simulink model "sdl_testbed"  (R2022b)
settings: Solver=VariableStepAuto  StartTime=0.0  StopTime=5  RelTol=1e-3  AbsTol=1e-3  EnableMultiTasking=on
PreLoadFcn:
  | MFormulaCoeff.DryTarmac = [10 1.9 1 0.97];
  | MFormulaCoeff.WetTarmac = [12 2.3 0.82 1];
  | MFormulaCoeff.Snow         = [5 2 0.3 1];
  | MFormulaCoeff.Ice            = [4 2 0.1 1];
libraries: sdl_lib x22, nesl_utility x9, fl_ps_legacy_lib x5, fl_lib x4, simulink x1
(part 1 of 3)
CloseFcn:
  | try,close(h1_sdl_vehicle_4wd_testbed),end
  | clear h1_sdl_vehicle_4wd_testbed
  | try,close(h2_sdl_vehicle_4wd_testbed),end
  | clear h2_sdl_vehicle_4wd_testbed
  | try,close(h3_sdl_vehicle_4wd_testbed),end
  | clear h3_sdl_vehicle_4wd_testbed
  | 
  | clear simlog_sdl_vehicle_4wd_testbed
  | clear logsout_sdl_vehicle_4wd_testbed
Description:
  | Four-Wheel Drive Testbed
settings Model: PacingRate=0.110000  Creator=The MathWorks, Inc.  LastModifiedBy=jc790999
settings SolverCC: AutoScaleAbsTol=off  MaxConsecutiveMinStep=2  AlgebraicLoopSolver=TrustRegion
settings DataIOCC: LimitDataPoints=on  MaxDataPoints=10000  SaveTime=off  ReturnWorkspaceOutputs=off  SignalLoggingName=logsout_sdl_vehicle_4wd_testbed
settings OptimizationCC: LifeSpan=inf
settings DebuggingCC: UnconnectedInputMsg=warning  UnconnectedOutputMsg=warning  UnconnectedLineMsg=warning  SFUnexpectedBacktrackingDiag=warning  SFNoUnconditionalDefaultTransitionDiag=warning  SFExecutionAtInitializationDiag=none  SFMachineParentedDataDiag=warning  ArithmeticOperatorsInVariantConditions=warning
settings HardwareCC: ProdBitPerPointer=32  ProdBitPerSizeT=32  ProdBitPerPtrDiffT=32  ProdLargestAtomicFloat=None  ProdIntDivRoundTo=Undefined  ProdEndianess=Unspecified  ProdWordSize=32  ProdHWDeviceType=32-bit Generic
settings ModelReferenceCC: EnableRefExpFcnMdlSchedulingChecks=on  PropagateSignalLabelsOutOfModel=off
settings SFSimCC: SimUseLocalCustomCode=off  CustomCodeUndefinedFunction=UseInterfaceOnly
settings RTWCC: RTWUseLocalCustomCode=off  DLArmComputeVersion=19.05
settings CodeAppCC: StateflowObjectComments=on
settings GRTTargetCC: TargetLangStandard=C89/C90 (ANSI)
settings ConfigComp: CovMetricSettings=dw  CovSaveCumulativeToWorkspaceVar=on  CovSaveSingleToWorkspaceVar=on  CovExternalEMLEnable=off  CovSFcnEnable=off
settings SimscapeCC: SimscapeLogType=all  SimscapeLogSimulationStatistics=on  SimscapeLogName=simlog_sdl_vehicle_4wd_testbed  SimscapeLogDataHistory=10000

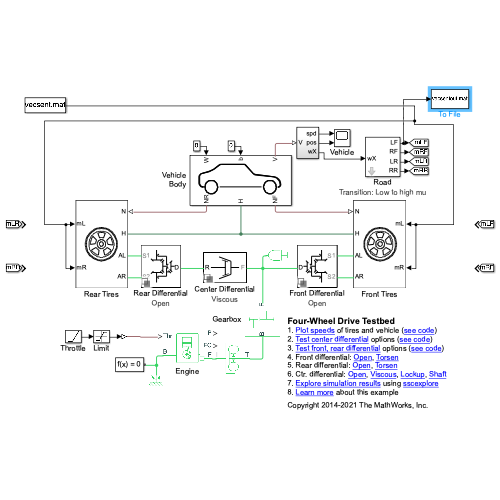
[thumbnail: Simulink's stored preview of the top-level diagram]
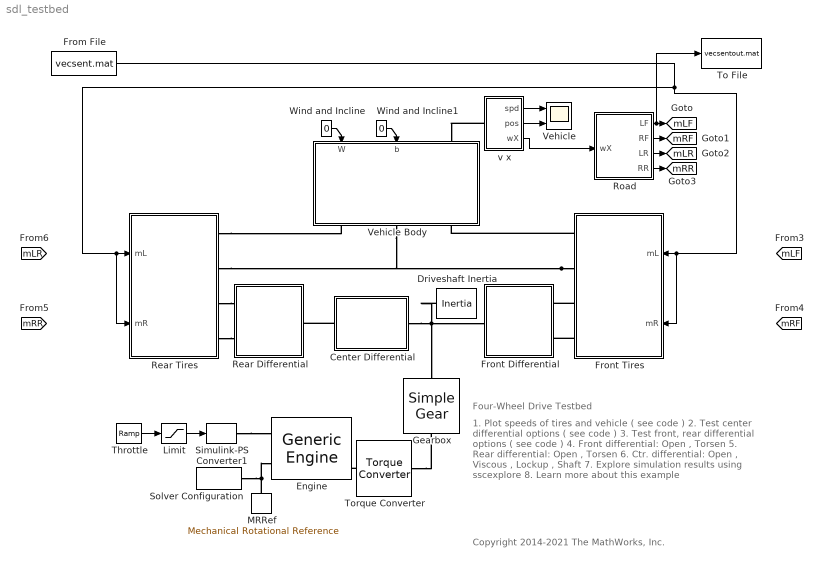
== system sdl_testbed ==
  note: Four-Wheel Drive Testbed
  note: 1. Plot speeds of tires and vehicle ( see code )
      | 2. Test center differential options ( see code )
      | 3. Test front, rear differential options ( see code )
      | 4. Front differential: Open , Torsen
      | 5. Rear differential: Open , Torsen
      | 6. Ctr. differential: Open , Viscous , Lockup , Shaft
      | 7. Explore simulation results using sscexplore
      | 8. Learn more about this example
  note: Copyright 2014-2021 The MathWorks, Inc.
  Center Differential : Subsystem  Variant=on  VariantControlMode=label  LabelModeActiveChoice=Viscous
      settings: AttributesFormatString=%<ActiveVariant>
      mask Display:
      | blk = find_system(gcbh, 'SearchDepth', 1, 'Parent', gcb, 'VariantObject', get_param(gcb,'activevariant'));
      | eval(get_param(blk, 'MaskDisplay'));
  Driveshaft Inertia : fl_lib/Mechanical/Rotational Elements/Inertia  inertia=12 kg*m^2  num_ports=foundation.enum.numPorts2.one  w_specify=off  w_priority=High  w=0 rpm  w_nominal_specify=off  w_nominal_unit=rad/s  w_nominal_value=1  t_specify=off  t_priority=High  t=0 N*m  t_nominal_specify=off  t_nominal_unit=N*m  t_nominal_value=1
  Engine : sdl_lib/Engines & Motors/Generic Engine  input_type=sdl.enum.GenericEngineInputType.NormalizedThrottle  model_parameterization=1  engine_type=1  Trq_max=380 N*m  w_Trq_max=4300 rpm  P_max=150e3 W  w_P_max=4500 rpm  w_max=6000 rpm  w_min=500 rpm  w_tab=[ 500 1000 2e+3 3e+3 4e+3 5e+3 6e+3 7e+3 ] rpm  trq_tab=[ 380 380 380 380 350 280 200 80 ] N*m  pwr_tab=[ 2e+4 4e+4 7.8e+4 1.2e+5 1.45e+5 1.48e+5 1.25e+5 6e+4 ] W  interp_method=simscape.enum.interpolation.linear  w_thr=100 rpm  model_inertia=1  inertia=0.2 kg*m^2  initial_velocity=800 rpm  model_time_constant=0  time_constant=0.2 s  initial_normalized_throttle=0  fc_model=0  fc_per_rev=25 mg/rev  fc_w_tab=[ 1000 2e+3 3e+3 4e+3 5e+3 6e+3 ] rpm  fc_trq_tab=[ 0 80 160 200 240 320 360 400 ] N*m  fc_tab=[ 0.5 0.9 1.4 1.6 1.9 2.7 3.4 4.4; 1 1.7 2.7 3.1 3.6 5 6 7.4; 1.4 2.7 4 4.8 5.6 7.5 8.5 10.5; 2 3.6 5.8 6.7 8 10.4 11.7 13.3; 2.5 4.8 7.9 9.4 10.8 14 16.2 18.6; 3.1 6 10.3 11.9 13.8 18.4 22 26.5 ] g/s  bmep_tab=[ 0 250 500 625 750 1000 1.15e+3 1.25e+3 ] kPa  bsfc_tab=[ 410 380 300 280 270 290 320 380; 410 370 290 270 260 270 285 320; 415 380 290 275 265 270 270 300; 420 390 310 290 285 280 280 285; 430 410 340 320 310 300 310 320; 450 430 370 340 330 330 350 380 ] g/hr/kW  fc_interp_method=simscape.enum.interpolation.linear  displaced_volume=400 cm^3  rev_per_cycle=2  idle_speed=0  idle_speed_reference=1000 rpm  tau_controller=1 s  idle_w_thr=1 rpm  redline=0  redline_speed=5000 rpm  tau_redline=1 s  redline_w_thr=1 rpm
      settings: InternalSimscapePortConfiguration="{\"Bottom\":[],\"Left\":[{\"id\":\"ThrNorm\",\"label\":\"Thr\",\"type\":\"input\"},{\"id\":\"B\",\"label\":\"B\",\"type\":\"foundation.mechanical.rotational.rotational\"}],\"Right\":[{\"id\":\"P\",\"label\":\"P\",\"type\":\"output\"},{\"id\":\"FC\",\"label\":\"FC\",\"type\":\"output\"},{\"id\":\"F\",\"label\":\"F\",\"type\":\"foundation.mechanical.rotational.rotational\"}],\"Top\":[]}"
  From File : FromFile  FileName=vecsent.mat  SampleTime=0
  Front Differential : Subsystem  Variant=on  VariantControlMode=label  LabelModeActiveChoice=Open
      settings: AttributesFormatString=%<ActiveVariant>
      mask Display:
      | blk = find_system(gcbh, 'SearchDepth', 1, 'Parent', gcb, 'VariantObject', get_param(gcb,'activevariant'));
      | eval(get_param(blk, 'MaskDisplay'));
  Front Tires : Subsystem
      mask Display:
      | plot([199.740630080105;207.645625381422;215.666495494822;223.725995056458;231.746506679781;239.614636200368], [285.533592122614;287.104128914395;287.892278108498;287.890449397339;287.098660392404;285.533592122614])
      | plot([182.29422131887;191.284049604609;200.547323621308;209.994832976365;219.535592990157;229.077720928241;238.529320882316;247.799368778054;256.798588986696;257.061044961602], [327.86290499758;331.09432156677;333.429020721321;334.844518032099;335.327181486212;334.872362770745;333.484442038558;331.176785725016;327.971617821912;327.86290499758])
      | plot([182.293066754937;199.741297401488], [327.862962149084;285.533680580556])
      | plot([239.613968878984;257.062199525535], [285.533680580556;327.862962149084])
      | plot([161.12998329239;162.078783791624;163.80431860203;166.28996988011;169.511799445263;173.438779317544;173.475674844307], [230.482414304504;238.453500201144;246.293204428793;253.926026350122;261.278457717503;268.279690597622;268.338450605791])
      | plot([115.521208412501;115.19363189143;115.795069625231;117.319729439748;119.752928027503;123.071232355974;127.242685340509;132.227113608518;137.976514391014;138.639091794056], [226.950718692202;236.412705455625;245.861238280392;255.205322630308;264.354969865087;273.222063880151;281.72120971289;289.770555942828;297.29258296555;298.068153121848])
      | plot([115.523664280772;161.128425970674], [226.952978409827;230.480418540537])
      | plot([173.474466428161;138.640995137393], [268.337409943342;298.068691045046])
      | plot([197.791294323752;190.505905487348;183.583957764389;177.092113295368;171.092892091325;165.644069931963;165.540704869119], [173.730032993176;177.080059057945;181.128046811489;185.835011918887;191.155623733067;197.038641853715;197.162104079289])
      | plot([187.018154556423;177.935574592276;169.151745387891;160.751260020237;152.815019755577;145.419454926048;138.635788863788;132.529351981303;127.158952603892;126.547993304079], [129.256249226993;131.857994736568;135.337460645285;139.661137794374;144.787386809327;150.666839109836;157.242872356214;164.45215575347;172.225259961496;173.223046112601])
      | plot([187.017316929996;197.78860732913], [129.25548478961;173.726426437497])
      | plot([165.537726134062;126.546914689243], [197.158707305789;173.222506418824])
      | plot([269.470357644972;273.38551933114;276.602305486856;279.089736702965;280.82385765709;281.787967816474;281.81616724833], [262.922159053497;255.989463868491;248.706398553292;241.143103008215;233.372415903877;225.469173204983;225.06588742066])
      | plot([304.431346528147;310.265227080294;315.332070863713;319.583081402952;322.977319142679;325.482095717982;327.073288761189;327.735574213461;327.462573903851;327.423015855416], [292.655530476138;285.116593543042;277.042138363134;268.509926353743;259.602127380701;250.404528417616;241.005707370423;231.496180023723;221.967528324303;221.475771485887])
      | plot([304.430681280792;269.471229985356], [292.651550844312;262.920269742608])
      | plot([281.817270442843;327.422032132745], [225.063278339803;221.472848206758])
      | plot([274.506490288884;269.03580586378;263.012187571475;256.493646148968;249.542958713556;242.227064184873;242.193171590222], [197.094155985096;191.184202827407;185.838928552521;181.109811073729;177.042394377551;173.675849910247;173.662235378073])
      | plot([313.374602600377;308.147922202874;302.181086731703;295.531560074253;288.263380807238;280.446545470191;272.156334460522;263.472587042146;254.478932449722;252.966160341391], [173.157457637183;165.349405231175;158.09125499764;151.452906891035;145.498291832517;140.284756020223;135.862508654033;132.274138393531;129.554203205929;129.189658564058])
      | plot([313.375261612236;274.510430172086], [173.15951641649;197.095717303455])
      | plot([242.196558974683;252.967849373817], [173.663436435163;129.192494787276])
      | plot([371.389053761959;370.658673461755;368.474566522701;364.857767088574;359.843106915069;353.478879920948;345.826377091206;336.959296211375;326.963032117569;315.933854297525;303.977979762811;291.210550120943;277.754522698759;263.739486396147;249.3004136741;234.576360696131;219.709128141403;204.841895586676;190.117842608706;175.678769886659;161.663733584047;148.207706161863;135.440276519995;123.484401985281;112.455224165237;102.458960071431;93.5918791916006;85.939376361858;79.5751493677372;74.5604891942319;70.9436897601051;68.7595828210511;68.0292025208473;68.7595828210511;70.9436897601053;74.5604891942321;79.5751493677375;85.9393763618583;93.5918791916009;102.458960071431;112.455224165237;123.484401985282;135.440276519995;148.207706161863;161.663733584048;175.67876988666;190.117842608707;204.841895586676;219.709128141403;234.576360696131;249.3004136741;263.739486396147;277.754522698759;291.210550120943;303.977979762811;315.933854297525;326.963032117569;336.959296211375;345.826377091205;353.478879920948;359.843106915069;364.857767088574;368.474566522701;370.658673461755;371.389053761959;371.389053761959;371.389053761959], [228.149788454175;213.282555899448;198.558502921478;184.119430199431;170.104393896819;156.648366474635;143.880936832767;131.925062298053;120.895884478009;110.899620384203;102.032539504372;94.3800366746299;88.0158096805091;83.0011495070038;79.3843500728769;77.2002431338229;76.4698628336191;77.2002431338229;79.3843500728769;83.0011495070038;88.0158096805092;94.38003667463;102.032539504373;110.899620384203;120.895884478009;131.925062298053;143.880936832767;156.648366474635;170.104393896819;184.119430199431;198.558502921479;213.282555899448;228.149788454175;243.017021008903;257.741073986872;272.180146708919;286.195183011531;299.651210433715;312.418640075584;324.374514610297;335.403692430341;345.399956524147;354.267037403978;361.91954023372;368.283767227841;373.298427401346;376.915226835473;379.099333774527;379.829714074731;379.099333774527;376.915226835473;373.298427401346;368.283767227841;361.91954023372;354.267037403978;345.399956524147;335.403692430341;324.374514610297;312.418640075583;299.651210433715;286.195183011531;272.180146708919;257.741073986872;243.017021008903;228.149788454176;228.149788454175;228.149788454175])
      | plot([363.45231346786;362.760150741504;360.690328467866;357.26278016692;352.510515002494;346.479299885972;339.227218715925;330.824112998412;321.350909235096;310.898839556798;299.568563108203;287.46919664527;274.717263681223;261.435572301422;247.752032454366;233.798424108965;219.709128141403;205.619832173842;191.666223828441;177.982683981384;164.700992601583;151.949059637537;139.849693174603;128.519416726008;118.067347047711;108.594143284395;100.191037566881;92.9389563968342;86.9077412803127;82.1554761158862;78.7279278149405;76.6581055413021;75.9659428149462;76.6581055413021;78.7279278149406;82.1554761158864;86.907741280313;92.9389563968345;100.191037566881;108.594143284395;118.067347047711;128.519416726009;139.849693174604;151.949059637537;164.700992601584;177.982683981384;191.666223828441;205.619832173842;219.709128141403;233.798424108965;247.752032454366;261.435572301422;274.717263681223;287.46919664527;299.568563108203;310.898839556798;321.350909235095;330.824112998411;339.227218715925;346.479299885972;352.510515002493;357.26278016692;360.690328467866;362.760150741504;363.45231346786;363.45231346786;363.45231346786], [228.149788454175;214.060492486614;200.106884141213;186.423344294156;173.141652914355;160.389719950309;148.290353487375;136.96007703878;126.508007360483;117.034803597167;108.631697879653;101.379616709606;95.3484015930846;90.596136428658;87.1685881277123;85.0987658540739;84.406603127718;85.0987658540739;87.1685881277124;90.5961364286582;95.3484015930846;101.379616709606;108.631697879653;117.034803597167;126.508007360483;136.960077038781;148.290353487376;160.389719950309;173.141652914355;186.423344294156;200.106884141213;214.060492486614;228.149788454175;242.239084421737;256.192692767138;269.876232614194;283.157923993995;295.909856958042;308.009223420975;319.33949986957;329.791569547868;339.264773311184;347.667879028697;354.919960198744;360.951175315265;365.703440479692;369.130988780638;371.200811054276;371.892973780632;371.200811054276;369.130988780638;365.703440479692;360.951175315265;354.919960198744;347.667879028697;339.264773311184;329.791569547868;319.33949986957;308.009223420975;295.909856958042;283.157923993995;269.876232614194;256.192692767138;242.239084421737;228.149788454176;228.149788454175;228.149788454175])
      | plot([261.408509686589;261.209838965396;260.615740109466;259.631934615548;258.267897068353;256.536763895118;254.455206854636;252.043272479101;249.324189015046;246.324142722634;243.072025687652;239.599157574934;235.93898400287;232.126754443812;228.199182752392;224.194093591025;220.150058157742;216.106022724459;212.100933563092;208.173361871672;204.361132312614;200.70095874055;197.228090627832;193.97597359285;190.975927300438;188.256843836383;185.844909460848;183.763352420366;182.032219247131;180.668181699936;179.684376206018;179.090277350088;178.891606628895;179.090277350088;179.684376206019;180.668181699936;182.032219247131;183.763352420366;185.844909460848;188.256843836383;190.975927300438;193.97597359285;197.228090627833;200.70095874055;204.361132312614;208.173361871672;212.100933563092;216.106022724459;220.150058157742;224.194093591025;228.199182752392;232.126754443812;235.93898400287;239.599157574934;243.072025687652;246.324142722634;249.324189015046;252.043272479101;254.455206854636;256.536763895118;258.267897068353;259.631934615548;260.615740109465;261.209838965396;261.408509686589;261.408509686589], [229.220618493855;225.176583060572;221.171493899205;217.243922207785;213.431692648727;209.771519076663;206.298650963945;203.046533928963;200.046487636551;197.327404172496;194.915469796961;192.833912756479;191.102779583244;189.738742036049;188.754936542131;188.160837686201;187.962166965008;188.160837686201;188.754936542131;189.738742036049;191.102779583244;192.833912756479;194.915469796961;197.327404172496;200.046487636551;203.046533928963;206.298650963945;209.771519076663;213.431692648727;217.243922207785;221.171493899205;225.176583060572;229.220618493855;233.264653927138;237.269743088505;241.197314779925;245.009544338983;248.669717911047;252.142586023765;255.394703058747;258.394749351159;261.113832815214;263.525767190749;265.607324231231;267.338457404466;268.702494951661;269.686300445579;270.280399301509;270.479070022702;270.280399301509;269.686300445579;268.702494951661;267.338457404466;265.607324231231;263.525767190749;261.113832815214;258.394749351159;255.394703058747;252.142586023765;248.669717911047;245.009544338983;241.197314779925;237.269743088505;233.264653927139;229.220618493855;229.220618493855])
      | plot([240.243868902326;240.144988512846;239.849299616612;239.359649859334;238.680754835845;237.819152676342;236.783141080621;235.58269740669;234.229382583359;232.736229772174;231.117618850946;229.38913792767;227.56743321852;225.670048735692;223.715257328969;221.721884708198;219.709128141403;217.696371574609;215.702998953837;213.748207547115;211.850823064286;210.029118355137;208.30063743186;206.682026510633;205.188873699447;203.835558876116;202.635115202186;201.599103606465;200.737501446962;200.058606423472;199.568956666194;199.27326776996;199.174387380481;199.27326776996;199.568956666194;200.058606423472;200.737501446962;201.599103606465;202.635115202186;203.835558876116;205.188873699447;206.682026510633;208.30063743186;210.029118355137;211.850823064286;213.748207547115;215.702998953837;217.696371574609;219.709128141403;221.721884708198;223.715257328969;225.670048735692;227.56743321852;229.38913792767;231.117618850946;232.736229772174;234.229382583359;235.58269740669;236.783141080621;237.819152676342;238.680754835845;239.359649859334;239.849299616612;240.144988512846;240.243868902326;240.243868902326], [230.66938854754;228.656631980745;226.663259359974;224.708467953251;222.811083470423;220.989378761273;219.260897837997;217.642286916769;216.149134105584;214.795819282253;213.595375608322;212.559364012601;211.697761853098;211.018866829609;210.529217072331;210.233528176097;210.134647786617;210.233528176097;210.529217072331;211.018866829609;211.697761853098;212.559364012601;213.595375608322;214.795819282253;216.149134105584;217.642286916769;219.260897837997;220.989378761273;222.811083470423;224.708467953251;226.663259359974;228.656631980745;230.66938854754;232.682145114334;234.675517735106;236.630309141828;238.527693624657;240.349398333806;242.077879257083;243.69649017831;245.189642989496;246.542957812827;247.743401486757;248.779413082478;249.641015241981;250.319910265471;250.809560022749;251.105248918983;251.204129308462;251.105248918983;250.809560022749;250.319910265471;249.641015241981;248.779413082478;247.743401486757;246.542957812827;245.189642989496;243.69649017831;242.077879257083;240.349398333806;238.527693624657;236.630309141828;234.675517735106;232.682145114334;230.66938854754;230.66938854754])
      | plot([339.327142573893;338.751149139472;337.02871596785;334.17643103205;330.22176339522;325.202798668544;319.167872225986;312.175103708213;304.291837298687;295.593993162365;286.165336293004;276.096669810484;265.484960477125;254.432404854758;243.045445095968;231.433743847976;219.709128141403;207.98451243483;196.372811186839;184.985851428048;173.933295805681;163.321586472322;153.252919989803;143.824263120442;135.126418984119;127.243152574594;120.250384056821;114.215457614262;109.196492887586;105.241825250756;102.389540314956;100.667107143335;100.091113708913;100.667107143335;102.389540314956;105.241825250756;109.196492887586;114.215457614262;120.250384056821;127.243152574594;135.12641898412;143.824263120442;153.252919989803;163.321586472323;173.933295805681;184.985851428048;196.372811186839;207.984512434831;219.709128141403;231.433743847976;243.045445095968;254.432404854758;265.484960477125;276.096669810484;286.165336293004;295.593993162365;304.291837298687;312.175103708212;319.167872225986;325.202798668544;330.22176339522;334.17643103205;337.02871596785;338.751149139472;339.327142573893;339.327142573893;339.327142573893], [228.149788454175;216.425172747602;204.813471499611;193.42651174082;182.373956118453;171.762246785094;161.693580302574;152.264923433213;143.567079296891;135.683812887366;128.691044369592;122.656117927034;117.637153200358;113.682485563528;110.830200627728;109.107767456107;108.531774021685;109.107767456107;110.830200627728;113.682485563528;117.637153200358;122.656117927034;128.691044369592;135.683812887366;143.567079296891;152.264923433214;161.693580302575;171.762246785094;182.373956118453;193.42651174082;204.813471499611;216.425172747602;228.149788454175;239.874404160748;251.48610540874;262.87306516753;273.925620789897;284.537330123256;294.605996605776;304.034653475137;312.732497611459;320.615764020985;327.608532538758;333.643458981316;338.662423707992;342.617091344822;345.469376280622;347.191809452243;347.767802886665;347.191809452243;345.469376280622;342.617091344822;338.662423707992;333.643458981316;327.608532538758;320.615764020985;312.732497611459;304.034653475137;294.605996605776;284.537330123256;273.925620789897;262.87306516753;251.48610540874;239.874404160748;228.149788454176;228.149788454175;228.149788454175])
      | plot([-20;467.858916595578;467.858916595578;-20;-20], [623.528016805649;623.528016805649;-170;-170;623.528016805649])
  Gearbox : sdl_lib/Gears/Simple Gear  ratio=2  rotation_direction=3-2*(1)  friction_model=1  T_noload=0.1 N*m  T_nom=5 N*m  efficiency_nom=0.8  efficiency=0.8  temperature_TLU=[ 280 300 320 ] K  load_TLU=[ 1 5 10 ] N*m  efficiency_TLU=[ 0.95 0.9 0.85 ]  efficiency_TLU2=[ 0.85 0.8 0.75; 0.95 0.9 0.85; 0.85 0.8 0.7 ]  w_thr=0.01 rad/s  pwr_thr=0.001 W  backlash_model=sdl.enum.backlashModel.Off  backlash_distance=1e-3 mm  x0=0 mm  r_base=0.1 m  hardstop_model=simscape.enum.hardstop.smooth  transition=1e-4 mm  backlash_stiffness=1e7 N/m  backlash_damping=1e6 N*s/m  e=0  v_tol=0.001 m/s  mu_visc=[ 0 0 ] N*m/(rad/s)  enable_faults=simscape.enum.onoff.off  efficiency_fault=0.05  external_fault=simscape.enum.onoff.off  temporal_fault=simscape.enum.onoff.off  fault_time=5 s  fault_angles=pi / 12 rad  report_fault=(1)-1  thermal_mass=50 J/K  temperature_specify=off  temperature_priority=High  temperature=300 K  temperature_nominal_specify=off  temperature_nominal_unit=K  temperature_nominal_value=1  x_backlash_specify=off  x_backlash_priority=None  x_backlash=0 mm  x_backlash_nominal_specify=off  x_backlash_nominal_unit=mm  x_backlash_nominal_value=1  f_hardstop_specify=off  f_hardstop_priority=None  f_hardstop=0 N  f_hardstop_nominal_specify=off  f_hardstop_nominal_unit=N  f_hardstop_nominal_value=1  v_backlash_specify=off  v_backlash_priority=None  v_backlash=0 m/s  v_backlash_nominal_specify=off  v_backlash_nominal_unit=m/s  v_backlash_nominal_value=1
  Limit : Saturate  UpperLimit=0.4  LowerLimit=0
  MRRef : fl_lib/Mechanical/Rotational Elements/Mechanical Rotational Reference
  Rear Differential : Subsystem  Variant=on  VariantControlMode=label  LabelModeActiveChoice=Open
      settings: AttributesFormatString=%<ActiveVariant>
      mask Display:
      | blk = find_system(gcbh, 'SearchDepth', 1, 'Parent', gcb, 'VariantObject', get_param(gcb,'activevariant'));
      | eval(get_param(blk, 'MaskDisplay'));
  Rear Tires : Subsystem
      mask Display:
      | plot([199.740630080105;207.645625381422;215.666495494822;223.725995056458;231.746506679781;239.614636200368], [285.533592122614;287.104128914395;287.892278108498;287.890449397339;287.098660392404;285.533592122614])
      | plot([182.29422131887;191.284049604609;200.547323621308;209.994832976365;219.535592990157;229.077720928241;238.529320882316;247.799368778054;256.798588986696;257.061044961602], [327.86290499758;331.09432156677;333.429020721321;334.844518032099;335.327181486212;334.872362770745;333.484442038558;331.176785725016;327.971617821912;327.86290499758])
      | plot([182.293066754937;199.741297401488], [327.862962149084;285.533680580556])
      | plot([239.613968878984;257.062199525535], [285.533680580556;327.862962149084])
      | plot([161.12998329239;162.078783791624;163.80431860203;166.28996988011;169.511799445263;173.438779317544;173.475674844307], [230.482414304504;238.453500201144;246.293204428793;253.926026350122;261.278457717503;268.279690597622;268.338450605791])
      | plot([115.521208412501;115.19363189143;115.795069625231;117.319729439748;119.752928027503;123.071232355974;127.242685340509;132.227113608518;137.976514391014;138.639091794056], [226.950718692202;236.412705455625;245.861238280392;255.205322630308;264.354969865087;273.222063880151;281.72120971289;289.770555942828;297.29258296555;298.068153121848])
      | plot([115.523664280772;161.128425970674], [226.952978409827;230.480418540537])
      | plot([173.474466428161;138.640995137393], [268.337409943342;298.068691045046])
      | plot([197.791294323752;190.505905487348;183.583957764389;177.092113295368;171.092892091325;165.644069931963;165.540704869119], [173.730032993176;177.080059057945;181.128046811489;185.835011918887;191.155623733067;197.038641853715;197.162104079289])
      | plot([187.018154556423;177.935574592276;169.151745387891;160.751260020237;152.815019755577;145.419454926048;138.635788863788;132.529351981303;127.158952603892;126.547993304079], [129.256249226993;131.857994736568;135.337460645285;139.661137794374;144.787386809327;150.666839109836;157.242872356214;164.45215575347;172.225259961496;173.223046112601])
      | plot([187.017316929996;197.78860732913], [129.25548478961;173.726426437497])
      | plot([165.537726134062;126.546914689243], [197.158707305789;173.222506418824])
      | plot([269.470357644972;273.38551933114;276.602305486856;279.089736702965;280.82385765709;281.787967816474;281.81616724833], [262.922159053497;255.989463868491;248.706398553292;241.143103008215;233.372415903877;225.469173204983;225.06588742066])
      | plot([304.431346528147;310.265227080294;315.332070863713;319.583081402952;322.977319142679;325.482095717982;327.073288761189;327.735574213461;327.462573903851;327.423015855416], [292.655530476138;285.116593543042;277.042138363134;268.509926353743;259.602127380701;250.404528417616;241.005707370423;231.496180023723;221.967528324303;221.475771485887])
      | plot([304.430681280792;269.471229985356], [292.651550844312;262.920269742608])
      | plot([281.817270442843;327.422032132745], [225.063278339803;221.472848206758])
      | plot([274.506490288884;269.03580586378;263.012187571475;256.493646148968;249.542958713556;242.227064184873;242.193171590222], [197.094155985096;191.184202827407;185.838928552521;181.109811073729;177.042394377551;173.675849910247;173.662235378073])
      | plot([313.374602600377;308.147922202874;302.181086731703;295.531560074253;288.263380807238;280.446545470191;272.156334460522;263.472587042146;254.478932449722;252.966160341391], [173.157457637183;165.349405231175;158.09125499764;151.452906891035;145.498291832517;140.284756020223;135.862508654033;132.274138393531;129.554203205929;129.189658564058])
      | plot([313.375261612236;274.510430172086], [173.15951641649;197.095717303455])
      | plot([242.196558974683;252.967849373817], [173.663436435163;129.192494787276])
      | plot([371.389053761959;370.658673461755;368.474566522701;364.857767088574;359.843106915069;353.478879920948;345.826377091206;336.959296211375;326.963032117569;315.933854297525;303.977979762811;291.210550120943;277.754522698759;263.739486396147;249.3004136741;234.576360696131;219.709128141403;204.841895586676;190.117842608706;175.678769886659;161.663733584047;148.207706161863;135.440276519995;123.484401985281;112.455224165237;102.458960071431;93.5918791916006;85.939376361858;79.5751493677372;74.5604891942319;70.9436897601051;68.7595828210511;68.0292025208473;68.7595828210511;70.9436897601053;74.5604891942321;79.5751493677375;85.9393763618583;93.5918791916009;102.458960071431;112.455224165237;123.484401985282;135.440276519995;148.207706161863;161.663733584048;175.67876988666;190.117842608707;204.841895586676;219.709128141403;234.576360696131;249.3004136741;263.739486396147;277.754522698759;291.210550120943;303.977979762811;315.933854297525;326.963032117569;336.959296211375;345.826377091205;353.478879920948;359.843106915069;364.857767088574;368.474566522701;370.658673461755;371.389053761959;371.389053761959;371.389053761959], [228.149788454175;213.282555899448;198.558502921478;184.119430199431;170.104393896819;156.648366474635;143.880936832767;131.925062298053;120.895884478009;110.899620384203;102.032539504372;94.3800366746299;88.0158096805091;83.0011495070038;79.3843500728769;77.2002431338229;76.4698628336191;77.2002431338229;79.3843500728769;83.0011495070038;88.0158096805092;94.38003667463;102.032539504373;110.899620384203;120.895884478009;131.925062298053;143.880936832767;156.648366474635;170.104393896819;184.119430199431;198.558502921479;213.282555899448;228.149788454175;243.017021008903;257.741073986872;272.180146708919;286.195183011531;299.651210433715;312.418640075584;324.374514610297;335.403692430341;345.399956524147;354.267037403978;361.91954023372;368.283767227841;373.298427401346;376.915226835473;379.099333774527;379.829714074731;379.099333774527;376.915226835473;373.298427401346;368.283767227841;361.91954023372;354.267037403978;345.399956524147;335.403692430341;324.374514610297;312.418640075583;299.651210433715;286.195183011531;272.180146708919;257.741073986872;243.017021008903;228.149788454176;228.149788454175;228.149788454175])
      | plot([363.45231346786;362.760150741504;360.690328467866;357.26278016692;352.510515002494;346.479299885972;339.227218715925;330.824112998412;321.350909235096;310.898839556798;299.568563108203;287.46919664527;274.717263681223;261.435572301422;247.752032454366;233.798424108965;219.709128141403;205.619832173842;191.666223828441;177.982683981384;164.700992601583;151.949059637537;139.849693174603;128.519416726008;118.067347047711;108.594143284395;100.191037566881;92.9389563968342;86.9077412803127;82.1554761158862;78.7279278149405;76.6581055413021;75.9659428149462;76.6581055413021;78.7279278149406;82.1554761158864;86.907741280313;92.9389563968345;100.191037566881;108.594143284395;118.067347047711;128.519416726009;139.849693174604;151.949059637537;164.700992601584;177.982683981384;191.666223828441;205.619832173842;219.709128141403;233.798424108965;247.752032454366;261.435572301422;274.717263681223;287.46919664527;299.568563108203;310.898839556798;321.350909235095;330.824112998411;339.227218715925;346.479299885972;352.510515002493;357.26278016692;360.690328467866;362.760150741504;363.45231346786;363.45231346786;363.45231346786], [228.149788454175;214.060492486614;200.106884141213;186.423344294156;173.141652914355;160.389719950309;148.290353487375;136.96007703878;126.508007360483;117.034803597167;108.631697879653;101.379616709606;95.3484015930846;90.596136428658;87.1685881277123;85.0987658540739;84.406603127718;85.0987658540739;87.1685881277124;90.5961364286582;95.3484015930846;101.379616709606;108.631697879653;117.034803597167;126.508007360483;136.960077038781;148.290353487376;160.389719950309;173.141652914355;186.423344294156;200.106884141213;214.060492486614;228.149788454175;242.239084421737;256.192692767138;269.876232614194;283.157923993995;295.909856958042;308.009223420975;319.33949986957;329.791569547868;339.264773311184;347.667879028697;354.919960198744;360.951175315265;365.703440479692;369.130988780638;371.200811054276;371.892973780632;371.200811054276;369.130988780638;365.703440479692;360.951175315265;354.919960198744;347.667879028697;339.264773311184;329.791569547868;319.33949986957;308.009223420975;295.909856958042;283.157923993995;269.876232614194;256.192692767138;242.239084421737;228.149788454176;228.149788454175;228.149788454175])
      | plot([261.408509686589;261.209838965396;260.615740109466;259.631934615548;258.267897068353;256.536763895118;254.455206854636;252.043272479101;249.324189015046;246.324142722634;243.072025687652;239.599157574934;235.93898400287;232.126754443812;228.199182752392;224.194093591025;220.150058157742;216.106022724459;212.100933563092;208.173361871672;204.361132312614;200.70095874055;197.228090627832;193.97597359285;190.975927300438;188.256843836383;185.844909460848;183.763352420366;182.032219247131;180.668181699936;179.684376206018;179.090277350088;178.891606628895;179.090277350088;179.684376206019;180.668181699936;182.032219247131;183.763352420366;185.844909460848;188.256843836383;190.975927300438;193.97597359285;197.228090627833;200.70095874055;204.361132312614;208.173361871672;212.100933563092;216.106022724459;220.150058157742;224.194093591025;228.199182752392;232.126754443812;235.93898400287;239.599157574934;243.072025687652;246.324142722634;249.324189015046;252.043272479101;254.455206854636;256.536763895118;258.267897068353;259.631934615548;260.615740109465;261.209838965396;261.408509686589;261.408509686589], [229.220618493855;225.176583060572;221.171493899205;217.243922207785;213.431692648727;209.771519076663;206.298650963945;203.046533928963;200.046487636551;197.327404172496;194.915469796961;192.833912756479;191.102779583244;189.738742036049;188.754936542131;188.160837686201;187.962166965008;188.160837686201;188.754936542131;189.738742036049;191.102779583244;192.833912756479;194.915469796961;197.327404172496;200.046487636551;203.046533928963;206.298650963945;209.771519076663;213.431692648727;217.243922207785;221.171493899205;225.176583060572;229.220618493855;233.264653927138;237.269743088505;241.197314779925;245.009544338983;248.669717911047;252.142586023765;255.394703058747;258.394749351159;261.113832815214;263.525767190749;265.607324231231;267.338457404466;268.702494951661;269.686300445579;270.280399301509;270.479070022702;270.280399301509;269.686300445579;268.702494951661;267.338457404466;265.607324231231;263.525767190749;261.113832815214;258.394749351159;255.394703058747;252.142586023765;248.669717911047;245.009544338983;241.197314779925;237.269743088505;233.264653927139;229.220618493855;229.220618493855])
      | plot([240.243868902326;240.144988512846;239.849299616612;239.359649859334;238.680754835845;237.819152676342;236.783141080621;235.58269740669;234.229382583359;232.736229772174;231.117618850946;229.38913792767;227.56743321852;225.670048735692;223.715257328969;221.721884708198;219.709128141403;217.696371574609;215.702998953837;213.748207547115;211.850823064286;210.029118355137;208.30063743186;206.682026510633;205.188873699447;203.835558876116;202.635115202186;201.599103606465;200.737501446962;200.058606423472;199.568956666194;199.27326776996;199.174387380481;199.27326776996;199.568956666194;200.058606423472;200.737501446962;201.599103606465;202.635115202186;203.835558876116;205.188873699447;206.682026510633;208.30063743186;210.029118355137;211.850823064286;213.748207547115;215.702998953837;217.696371574609;219.709128141403;221.721884708198;223.715257328969;225.670048735692;227.56743321852;229.38913792767;231.117618850946;232.736229772174;234.229382583359;235.58269740669;236.783141080621;237.819152676342;238.680754835845;239.359649859334;239.849299616612;240.144988512846;240.243868902326;240.243868902326], [230.66938854754;228.656631980745;226.663259359974;224.708467953251;222.811083470423;220.989378761273;219.260897837997;217.642286916769;216.149134105584;214.795819282253;213.595375608322;212.559364012601;211.697761853098;211.018866829609;210.529217072331;210.233528176097;210.134647786617;210.233528176097;210.529217072331;211.018866829609;211.697761853098;212.559364012601;213.595375608322;214.795819282253;216.149134105584;217.642286916769;219.260897837997;220.989378761273;222.811083470423;224.708467953251;226.663259359974;228.656631980745;230.66938854754;232.682145114334;234.675517735106;236.630309141828;238.527693624657;240.349398333806;242.077879257083;243.69649017831;245.189642989496;246.542957812827;247.743401486757;248.779413082478;249.641015241981;250.319910265471;250.809560022749;251.105248918983;251.204129308462;251.105248918983;250.809560022749;250.319910265471;249.641015241981;248.779413082478;247.743401486757;246.542957812827;245.189642989496;243.69649017831;242.077879257083;240.349398333806;238.527693624657;236.630309141828;234.675517735106;232.682145114334;230.66938854754;230.66938854754])
      | plot([339.327142573893;338.751149139472;337.02871596785;334.17643103205;330.22176339522;325.202798668544;319.167872225986;312.175103708213;304.291837298687;295.593993162365;286.165336293004;276.096669810484;265.484960477125;254.432404854758;243.045445095968;231.433743847976;219.709128141403;207.98451243483;196.372811186839;184.985851428048;173.933295805681;163.321586472322;153.252919989803;143.824263120442;135.126418984119;127.243152574594;120.250384056821;114.215457614262;109.196492887586;105.241825250756;102.389540314956;100.667107143335;100.091113708913;100.667107143335;102.389540314956;105.241825250756;109.196492887586;114.215457614262;120.250384056821;127.243152574594;135.12641898412;143.824263120442;153.252919989803;163.321586472323;173.933295805681;184.985851428048;196.372811186839;207.984512434831;219.709128141403;231.433743847976;243.045445095968;254.432404854758;265.484960477125;276.096669810484;286.165336293004;295.593993162365;304.291837298687;312.175103708212;319.167872225986;325.202798668544;330.22176339522;334.17643103205;337.02871596785;338.751149139472;339.327142573893;339.327142573893;339.327142573893], [228.149788454175;216.425172747602;204.813471499611;193.42651174082;182.373956118453;171.762246785094;161.693580302574;152.264923433213;143.567079296891;135.683812887366;128.691044369592;122.656117927034;117.637153200358;113.682485563528;110.830200627728;109.107767456107;108.531774021685;109.107767456107;110.830200627728;113.682485563528;117.637153200358;122.656117927034;128.691044369592;135.683812887366;143.567079296891;152.264923433214;161.693580302575;171.762246785094;182.373956118453;193.42651174082;204.813471499611;216.425172747602;228.149788454175;239.874404160748;251.48610540874;262.87306516753;273.925620789897;284.537330123256;294.605996605776;304.034653475137;312.732497611459;320.615764020985;327.608532538758;333.643458981316;338.662423707992;342.617091344822;345.469376280622;347.191809452243;347.767802886665;347.191809452243;345.469376280622;342.617091344822;338.662423707992;333.643458981316;327.608532538758;320.615764020985;312.732497611459;304.034653475137;294.605996605776;284.537330123256;273.925620789897;262.87306516753;251.48610540874;239.874404160748;228.149788454176;228.149788454175;228.149788454175])
      | plot([-20;467.858916595578;467.858916595578;-20;-20], [623.528016805649;623.528016805649;-170;-170;623.528016805649])
  Road : Subsystem  mask(Testing Surface){road_condition=Transition: Low to high mu, surface_LF=0, surface_RF=0, surface_LR=0, surface_RR=0, surface_xpos=0}
      mask prompts: road_condition "Road Condition"; surface_LF "Surface LF"; surface_RF "Surface RF"; surface_LR "Surface LR"; surface_RR "Surface RR"; surface_xpos "Surface Position"
      mask help: Select surface for test. Specifies locations of high and low friction surface as a function of longitudinal distance for each tire.
      mask init:
      | if (road_condition==1)
      |     % Road: low coeff to high coeff
      |     surface_LF   = [4 1 1 4 4];
      |     surface_RF   = [4 1 1 4 4];
      |     surface_LR   = [4 1 1 4 4];
      |     surface_RR   = [4 1 1 4 4];
      |     surface_xpos = [-1 0 2.5 5 6];
      | elseif(road_condition==2)
      |     % Road: Split (low left side)
      |     surface_LF   = [1 1 1 1 1];
      |     surface_RF   = [4 4 4 4 4];
      |     surface_LR   = [1 1 1 1 1];
      |     surface_RR   = [4 4 4 4 4];
      |     surface_xpos = [-1 0 4.9 5 6];
      | end
      settings: AttributesFormatString=%<road_condition>
      mask TypeOptions road_condition: Transition: Low to high mu | Split: Low mu on left
  Simulink-PS Converter1 : nesl_utility/Simulink-PS Converter  PhysicalDomain=network_engine_domain  SubClassName=ps_input  LeftPortType=input  RightPortType=output  PseudoPeriodic=off  Frequencies=[]  NoiseDistribution=none  NoiseParameters=[]  Unit=1  AffineConversion=off  FilteringAndDerivatives=zero  SimscapeFilterOrder=1  InputFilterTimeConstant=.001  UdotUserProvided=0
  Solver Configuration : nesl_utility/Solver Configuration  PhysicalDomain=network_engine_domain  SubClassName=solver  LeftPortType=input  RightPortType=generic  Tones=[]  Harmonics=[]  SimulateNoise=off  Profile=off  UseLocalSampling=off  EnableSwitchedLinearOptims=on  FrequencyDomain=off  UseCCode=off  RelTol=0.001  AbsTol=1e-06  MinStep=1e-09  ToWorkspace=off  RevertToSquareIcSolve=off  NumHomotopyIterations=100  PhasorMode=off  PhasorModeNumHarmonics=1  ConsistencySolver=NEWTON_FTOL  IndexReductionMethod=DerivativeReplacement  DoDC=off  ResidualTolerance=1e-9  ConsistencyTolSource=GLOBAL  ConsistencyAbsTol=0.001  ConsistencyRelTol=0.001  ConsistencyTolFactor=0.001  UseLocalSolver=off  LocalSolverChoice=NE_BACKWARD_EULER_ADVANCER  ResolveIndetEquations=on  FunctionEvalNumThread=1  LocalSolverSampleTime=0.001  DoFixedCost=off  MaxNonlinIter=3  MaxModeIter=2  ComputeImpulses=off  ImpulseIterations=2  LinearAlgebra=auto  LinearAlgebraNumThread=0  EquationFormulation=NE_TIME_EF  DelaysMemoryBudget=1024  AutomaticFiltering=on  FilteringTimeConstant=0.001  PartitionStorageMethod=AS_NEEDED  PartitionMemoryBudget=1024  PartitionMethod=FAST
  Throttle : simulink/Sources/Ramp  slope=0.9/2  start=0  InitialOutput=0.02
  To File : ToFile  Filename=vecsentout.mat
  Torque Converter : sdl_lib/Couplings & Drives/Torque Converter  coast_mode_modeling=sdl.enum.torqueConverterContinuousTwomode.continuous  SR_drive_tlu=[0, .5, .6, .7, .8, .87, .92, .94, .96, .97, 1]  TR_drive_tlu=[2.232, 1.5462, 1.4058, 1.2746, 1.1528, 1.0732, 1.0192, 1, 1, 1, 1]  CF_drive_tlu=1e-4 * [.72558, .66322, .63463, .59042, .51331, .4144, .29287, .22444, .12186, .04386, 0] m*N/rpm^2  SR_coast_tlu=[0, .5, .6, .7, .8, .87, .92, .94, .96, .97, 1]  CF_coast_tlu=1e-4 * [.5079, .4643, .4442, .4133, .3593, .2901, .205, .1571, .0853, .0307, 0] m*N/rpm^2  iniMode=sdl.enum.torqueConverterInitialMode.drive  delta_w=1 rpm  n_vector=[0 0.50 0.60 0.70 0.80 0.87 0.92 0.94 0.96 0.97]  trq_vector=[2.2320 1.5462 1.4058 1.2746 1.1528 1.0732 1.0192 0.9983 0.9983 0.9983]  cf_vector_parameterization=1  cf_vector_reference_speed=1  cf_vector=[12.2938 12.8588 13.1452 13.6285 14.6163 16.2675 19.3503 22.1046 29.9986 50.00] (rad/s)/(N*m)^0.5  cf_vector_sq=1e-3*[ 6.616 6.048 5.787 5.384 4.681 3.779 2.671 2.047 1.111 0.400] N*m/(rad/s)^2  interp_method=1  extrap_method=1  model_lag=0  tau=0.02 s  initial_trq_ratio=0
      settings: InternalSimscapePortConfiguration="{\"Bottom\":[],\"Left\":[{\"id\":\"I\",\"label\":\"I\",\"type\":\"foundation.mechanical.rotational.rotational\"}],\"Right\":[{\"id\":\"T\",\"label\":\"T\",\"type\":\"foundation.mechanical.rotational.rotational\"}],\"Top\":[]}"
  Vehicle : Scope  NumInputPorts=2
  Vehicle Body : Subsystem
      mask Display:
      | color('white')
      | plot(-120,-70); plot(120,40);
      | color('black')
      | plot(sin(0:0.1:6*pi)*15-70,cos(0:0.1:6*pi)*15-30);
      | plot(sin(0:0.1:6*pi)*15+70,cos(0:0.1:6*pi)*15-30);
      | plot([-88 -95 -99 -99 -95 -75 -65 -50 -46 10 30 34 80 85 90 93 95 93 90 88],[-30 -28 -23 -5 0 5 10 20 21 21 0 -2 -7 -9 -13 -17 -25 -28 -30 -30])
      | plot([-88 -95 -99 -99 -95 -75 -65 -50 -46 10 30 34 80 85 90 93 95 93 90 88],[-30 -28 -23 -5 0 5 10 20 21 21 0 -2 -7 -9 -13 -17 -25 -28 -30 -30]-1)
      | plot([-88 -95 -99 -99 -95 -75 -65 -50 -46 10 30 34 80 85 90 93 95 93 90 88]+1,[-30 -28 -23 -5 0 5 10 20 21 21 0 -2 -7 -9 -13 -17 -25 -28 -30 -30])
      | plot([-50 50],[-30 -30])
  Wind and Incline : Constant  Value=0
  Wind and Incline1 : Constant  Value=0
  v x : Subsystem
  tag scope: mLF=global, mLR=global, mRF=global, mRR=global
  wires:
  Limit/1 -> Simulink-PS Converter1/1
  Throttle/1 -> Limit/1
  Wind and Incline/1 -> Vehicle Body/1(W)
  v x/1(spd) -> Vehicle/1
  v x/2(pos) -> Vehicle/2
  Wind and Incline1/1 -> Vehicle Body/2(b)
  Road/1(LF) -> To File/1, [mLF]
  Road/2(RF) -> [mRF]
  Road/3(LR) -> [mLR]
  Road/4(RR) -> [mRR]
  v x/3(wX) -> Road/1(wX)
  From File/1 -> Front Tires/2(mR), Front Tires/1(mL), Rear Tires/2(mR), Rear Tires/1(mL)
  connections:
  Center Differential/LConn1 -- Rear Differential/LConn1
  Driveshaft Inertia/LConn1 -- Gearbox/RConn1 -- Front Differential/LConn1 -- Center Differential/RConn1
  Torque Converter/RConn1 -- Gearbox/LConn1
  Simulink-PS Converter1/RConn1 -- Engine/LConn1
  MRRef/LConn1 -- Solver Configuration/RConn1 -- Engine/LConn2
  Torque Converter/LConn1 -- Engine/RConn3
  v x/LConn1 -- Vehicle Body/LConn1
  Front Tires/RConn1 -- Vehicle Body/RConn3
  Front Tires/RConn3 -- Front Differential/RConn1
  Front Tires/RConn4 -- Front Differential/RConn2
  Front Tires/RConn2 -- Rear Tires/RConn2 -- Vehicle Body/RConn2
  Rear Tires/RConn1 -- Vehicle Body/RConn1
  Rear Tires/RConn3 -- Rear Differential/RConn1
  Rear Tires/RConn4 -- Rear Differential/RConn2
